simulink model "flmpc_simulink"  (R2023a)
settings: Solver=ode1  StartTime=0.0  StopTime=inf  FixedStep=0.1  RelTol=1e-3
settings Model: Creator=pindiche  LastModifiedBy=bajdus

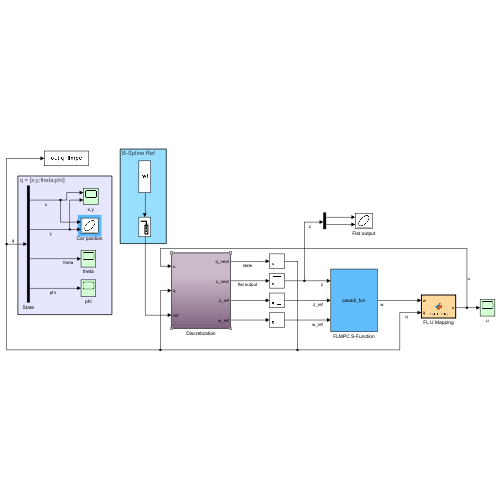
[thumbnail: Simulink's stored preview of the top-level diagram]
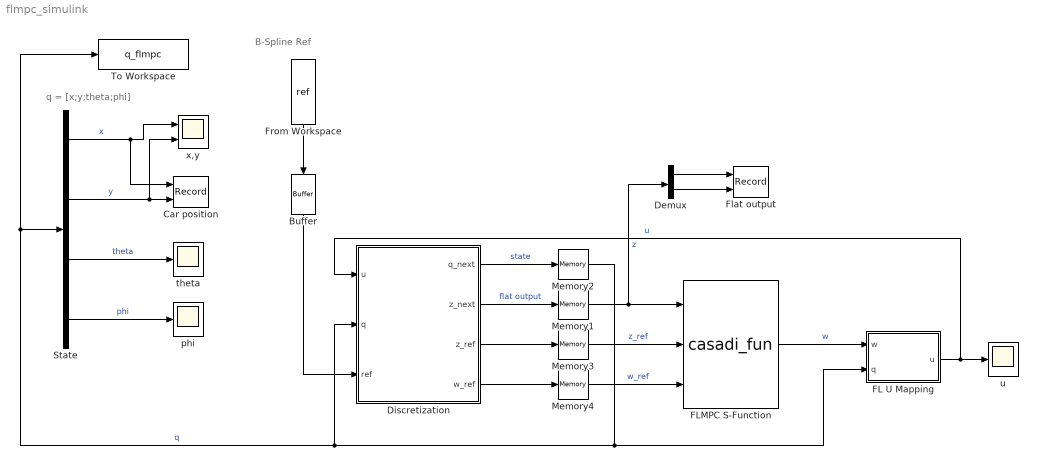
== system flmpc_simulink ==
  note: q = [x;y;theta;phi]
  note: B-Spline Ref
  Buffer : Buffer  N=54  OutputFrames=off
  Car position : Record  FileSettingsInternal="{\"entries\":[{\"content\":{\"excelSettings\":{\"content\":{},\"type\":\"Streamout.ExcelSettings\"}},\"type\":\"Streamout.FileSettingStorage\",\"uuid\":\"\"}],\"packageUris\":[\"http:\\/\\/schema.mathworks.com\\/mf0\\/streamout_blocks\\/R2020a\"],\"version\":\"1.0\"}"  Layout=[1 1]  SignalsInternal="{\"entries\":[{\"content\":{\"signals\":[{\"content\":{\"blockPath\":[],\"dimensions\":[1,1],\"domain\":\"\",\"lineColor\":\"#a2142f\",\"plots\":[1],\"port\":1,\"sid\":[\"\"],\"signalID\":2660,\"signalName\":\"x\"},\"type\":\"RecordBlkView.Signal\",\"uuid\":\"\"},{\"content\":{\"blockPath\":[],\"dimensions\":[1,1],\"domain\":\"\",\"lineColor\":\"#139fff\",\"plots\":[1],\"port\":2,\"sid\":[\"\"],\"signalID\":2664,\"signalName\":\"y\"},\"type\":\"RecordBlkView.Signal\",\"uuid\":\"\"}]},\"type\":\"RecordBlkView.InputSignals\",\"uuid\":\"\"}],\"packageUris\":[\"http:\\/\\/schema.mathworks.com\\/mf0\\/streamout_blocks\\/R2020a\"],\"version\":\"1.0\"}"  VisualizationBindings="{\"xyplotplugin\":{\"info\":[{\"series\":[{\"bindingParametersList\":[{\"parameter\":\"X-Axis\",\"signalID\":2660,\"signalName\":\"x\"},{\"parameter\":\"Y-Axis\",\"signalID\":2664,\"signalName\":\"y\"}],\"seriesID\":21245}],\"subplotID\":1}]}}"  CompatibilityTag=XY
  Demux : Demux  Outputs=2
  Discretization : Subsystem
  FL U Mapping : MATLAB Function  TreatAsAtomicUnit=on
  FLMPC S-Function : S-Function  FunctionName=casadi_fun  Parameters='flmpc_fun.casadi','flmpc_fun'  SFunctionDeploymentMode=off  EnableBusSupport=off
  Flat output : Record  FileSettingsInternal="{\"entries\":[{\"content\":{\"excelSettings\":{\"content\":{},\"type\":\"Streamout.ExcelSettings\"}},\"type\":\"Streamout.FileSettingStorage\",\"uuid\":\"\"}],\"packageUris\":[\"http:\\/\\/schema.mathworks.com\\/mf0\\/streamout_blocks\\/R2020a\"],\"version\":\"1.0\"}"  Layout=[1 1]  SignalsInternal="{\"entries\":[{\"content\":{\"signals\":[{\"content\":{\"blockPath\":[],\"dimensions\":[1,1],\"domain\":\"\",\"lineColor\":\"#a2142f\",\"plots\":[1],\"port\":1,\"sid\":[\"\"],\"signalID\":2668,\"signalName\":\"Demux:1\"},\"type\":\"RecordBlkView.Signal\",\"uuid\":\"\"},{\"content\":{\"blockPath\":[],\"dimensions\":[1,1],\"domain\":\"\",\"lineColor\":\"#139fff\",\"plots\":[1],\"port\":2,\"sid\":[\"\"],\"signalID\":2672,\"signalName\":\"Demux:2\"},\"type\":\"RecordBlkView.Signal\",\"uuid\":\"\"}]},\"type\":\"RecordBlkView.InputSignals\",\"uuid\":\"\"}],\"packageUris\":[\"http:\\/\\/schema.mathworks.com\\/mf0\\/streamout_blocks\\/R2020a\"],\"version\":\"1.0\"}"  VisualizationBindings="{\"xyplotplugin\":{\"info\":[{\"series\":[{\"bindingParametersList\":[{\"parameter\":\"X-Axis\",\"signalID\":2668,\"signalName\":\"Demux:1\"},{\"parameter\":\"Y-Axis\",\"signalID\":2672,\"signalName\":\"Demux:2\"}],\"seriesID\":18967}],\"subplotID\":1}]}}"  CompatibilityTag=XY
  From Workspace : FromWorkspace  VariableName=ref  SampleTime=0.1  ZeroCross=off
  Memory{1..4} (4 alike) : Memory
  State : Demux
  To Workspace : ToWorkspace  VariableName=q_flmpc  SaveFormat=Timeseries  SampleTime=-1
  phi : Scope
  theta : Scope
  u : Scope
  x,y : Scope  NumInputPorts=2
  wires:
  State/4 -> phi/1  "phi"
  State/3 -> theta/1  "theta"
  State/1 -> Car position/1, x,y/1  "x"
  State/2 -> Car position/2, x,y/2  "y"
  FL U Mapping/1(u) -> Discretization/1(u), u/1  "u"
  Memory1/1 -> Demux/1, FLMPC S-Function/1  "z"
  Discretization/1(q_next) -> Memory2/1  "state"
  Memory2/1 -> Discretization/2(q), To Workspace/1, State/1, FL U Mapping/2(q)  "q"
  FLMPC S-Function/1 -> FL U Mapping/1(w)  "w"
  Discretization/2(z_next) -> Memory1/1  "flat output"
  Demux/1 -> Flat output/1
  Demux/2 -> Flat output/2
  From Workspace/1 -> Buffer/1
  Buffer/1 -> Discretization/3(ref)
  Discretization/3(z_ref) -> Memory3/1
  Memory3/1 -> FLMPC S-Function/2  "z_ref"
  Discretization/4(w_ref) -> Memory4/1
  Memory4/1 -> FLMPC S-Function/3  "w_ref"

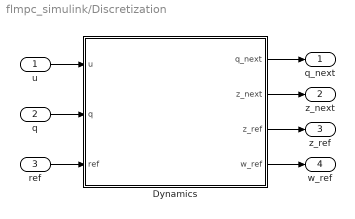
== system flmpc_simulink/Discretization ==
  u : Inport
  q : Inport  Port=2
  ref : Inport  Port=3
  Dynamics : MATLAB Function  TreatAsAtomicUnit=on
  q_next : Outport  PortDimensions=[4,1]
  z_next : Outport  Port=2  PortDimensions=[2,1]
  z_ref : Outport  Port=3  PortDimensions=[2,6]
  w_ref : Outport  Port=4  PortDimensions=[2,5]
  wires:
  u/1 -> Dynamics/1(u)
  q/1 -> Dynamics/2(q)
  Dynamics/2(z_next) -> z_next/1
  Dynamics/1(q_next) -> q_next/1
  ref/1 -> Dynamics/3(ref)
  Dynamics/3(z_ref) -> z_ref/1
  Dynamics/4(w_ref) -> w_ref/1

== matlab function flmpc_simulink/FL U Mapping ==
  data: w input; u output; q input
function u = mapping(w, q)

Delta = 0.35;
L = 0.256;
eta = [q(3); q(4)];
s1 = sin(eta(1)+eta(2)); c1 = cos(eta(1)+eta(2)); 
M = [cos(eta(1))-tan(eta(2))*(sin(eta(1))+Delta*s1/L), -Delta*s1;
     sin(eta(1))+tan(eta(2))*(cos(eta(1))+Delta*c1/L),  Delta*c1];

u = M^(-1) * w(:, 1);

end

== matlab function flmpc_simulink/Discretization/Dynamics ==
  data: u input; q_next output; q input; z_next output; ref input; z_ref output; w_ref output
function [q_next, z_next, z_ref, w_ref] = discrete_plant(u, q, ref)
    persistent idx z_ref_internal;

    if isempty(idx)
        idx = 1;
    end

    if isempty(z_ref_internal)
        z_ref_internal = zeros(2,1);
    end

    % Parameters
    Npred = 5;
    l = 0.256;
    L = l;
    Delta = 0.35;
    dt = 0.1;  
    
    %% Next flat output
    x = q(1);
    y = q(2);
    theta = q(3);
    phi = q(4);

    v = u(1); 
    omega = u(2);  

    % Discretized system dynamics
    x_next = x + dt * (v * cos(theta));  
    y_next = y + dt * (v * sin(theta)); 
    theta_next = theta + dt * (v / l * tan(phi));  
    phi_next = phi + dt * omega; 

    q_next = [x_next; y_next; theta_next; phi_next];
    z_next = [q_next(1)+L*cos(q_next(3))+Delta*cos(q_next(3)+q_next(4));
              q_next(2)+L*sin(q_next(3))+Delta*sin(q_next(3)+q_next(4))];

    %% Reference
    % spline
    ref = reshape(ref,[9,Npred+1]);
    xr = ref(2, :);
    yr = ref(3, :);
    dddxr = ref(4, :);
    dddyr = ref(5, :);
    ddxr = ref(6, :);
    ddyr = ref(7, :);
    dxr = ref(8, :);
    dyr = ref(9, :);

    % circle
    t = 0:dt:60;  
    alpha   = 5;
    beta    = 5;
    ang     = 0.2;
    xr = alpha*cos(ang*t);      dxr = -alpha*ang*sin(ang*t);    ddxr = -alpha*ang*ang*cos(ang*t);       dddxr = alpha*ang*ang*ang*sin(ang*t);
    yr = beta*sin(ang*t);       dyr = beta*ang*cos(ang*t);      ddyr = -beta*ang*ang*sin(ang*t);        dddyr = -beta*ang*ang*ang*cos(ang*t);

    Vr = sqrt(dxr.^2 + dyr.^2);
    omegar  = l * Vr .* ((dddyr.*dxr - dddxr.*dyr).*Vr.*Vr - 3 * (ddyr.*dxr - ddxr.*dyr) .* (dxr.*ddxr + dyr.*ddyr)) ...
              ./ (Vr.^6 + l*l*(ddyr.*dxr - ddxr.*dyr).^2);

    thetar = unwrap(atan2(dyr, dxr));
    phir = atan((l*(ddyr.*dxr - ddxr.*dyr)) ./ Vr.^3);
    
    % references predefined inside here
    q_ref = zeros(4, Npred + 1);
    z_ref = zeros(2, Npred + 1);
    w_ref = zeros(2, Npred);
    % ur    = zeros(2, Npred + 1);
    idx_end = min(idx + Npred, size(t,2));
    
    q_ref(1, :) = xr(idx:idx_end);
    q_ref(2, :) = yr(idx:idx_end);
    q_ref(3, :) = thetar(idx:idx_end);
    q_ref(4, :) = phir(idx:idx_end);

    % q_ref(1, :) = xr;
    % q_ref(2, :) = yr;
    % q_ref(3, :) = thetar;
    % q_ref(4, :) = phir;

    for k = 1:Npred+1
        z_ref(1, k) = q_ref(1,k) + L*cos(q_ref(3,k)) + Delta*cos(q_ref(3,k)+q_ref(4,k));
        z_ref(2, k) = q_ref(2,k) + L*sin(q_ref(3,k)) + Delta*sin(q_ref(3,k)+q_ref(4,k));
    end
    
    % ur(1,:) = Vr; 
    % ur(2,:) = omegar;
    ur = [Vr; omegar];

    wref = zeros(2, length(xr));
    len  = length(xr);
    for i = 1:len
        s1        = sin(thetar(i) + phir(i)); 
        c1        = cos(thetar(i) + phir(i));
        M         = [cos(thetar(i)) - tan(phir(i))*(sin(thetar(i)) + Delta*s1/l), -Delta*s1;
                     sin(thetar(i)) + tan(phir(i))*(cos(thetar(i)) + Delta*c1/l),  Delta*c1];
        wref(:,i) = M * ur(:,i);
    end
    w_ref(1,1:Npred) = wref(1, idx:idx_end-1);
    w_ref(2,1:Npred) = wref(2, idx:idx_end-1);
    % w_ref = wref(:, 1:Npred);
    idx = idx + 1;
end
